simulink library "amg_high_precision_rtc"  (R2015b)
settings: Solver=ode45  StartTime=0.0  StopTime=10.0  RelTol=1e-3
libraries: simulink x207, waijung_soft_i2c_lib x11, amg_high_precision_rtc x10
(part 2 of 5)

== system amg_high_precision_rtc/STM32F4/DS3231 Get Date/Convert ==
  In1 : Inport
  In2 : Inport  Port=2
  In3 : Inport  Port=3
  In4 : Inport  Port=4
  Enable : EnablePort  PropagateVarSize=During execution
  Convert 1 : Subsystem
  Convert 2 : Subsystem
  Convert 3 : Subsystem
  Data Type Conversion{,1..3} (4 alike) : DataTypeConversion  OutDataTypeStr=uint8
  Extract Bits : simulink/Logic and Bit Operations/Extract Bits  SystemSampleTime=-1  bitsToExtract=Range of bits  numBits=8  bitIdxRange=[0 3]  outScalingMode=Treat bit field as an integer
  Day : Outport
  Date : Outport  Port=2
  Month : Outport  Port=3
  Year : Outport  Port=4
  wires:
  In1/1 -> Extract Bits/1
  Extract Bits/1 -> Data Type Conversion/1
  Convert 1/1(Out1) -> Data Type Conversion1/1
  In2/1 -> Convert 1/1(In1)
  In3/1 -> Convert 2/1(In1)
  Convert 2/1(Out1) -> Data Type Conversion2/1
  In4/1 -> Convert 3/1(In1)
  Convert 3/1(Out1) -> Data Type Conversion3/1
  Data Type Conversion/1 -> Day/1
  Data Type Conversion1/1 -> Date/1
  Data Type Conversion2/1 -> Month/1
  Data Type Conversion3/1 -> Year/1

== system amg_high_precision_rtc/STM32F4/DS3231 Get Time/Convert ==
  In1 : Inport
  In2 : Inport  Port=2
  In3 : Inport  Port=3
  Enable : EnablePort  PropagateVarSize=During execution
  Convert Hour : Subsystem
  Convert Second/ Minute : Subsystem
  Demux : Demux  Outputs=2
  Mux : Mux  Inputs=2
  Hour : Outport
  Minute : Outport  Port=2
  Second : Outport  Port=3
  AM/PM : Outport  Port=4
  wires:
  In2/1 -> Mux/2
  In1/1 -> Mux/1
  Mux/1 -> Convert Second/ Minute/1(In1)
  Convert Second/ Minute/1(Out1) -> Demux/1
  Demux/1 -> Second/1
  Demux/2 -> Minute/1
  In3/1 -> Convert Hour/1(In1)
  Convert Hour/1(Hour) -> Hour/1
  Convert Hour/2(AM/PM) -> AM/PM/1

== system amg_high_precision_rtc/STM32F4/DS3231 Set Date/ConvertToBCD1 ==
  In1 : Inport
  Bitwise Operator : simulink/Logic and Bit Operations/Bitwise Operator  logicop=OR  UseBitMask=off  NumInputPorts=2  BitMask=bin2dec('11011001')  BitMaskRealWorld=Stored Integer
  Constant : Constant  Value=10  OutDataTypeStr=single
  Constant1 : Constant  Value=10  OutDataTypeStr=single
  Data Type Conversion : DataTypeConversion  OutDataTypeStr=single
  Data Type Conversion1 : DataTypeConversion  OutDataTypeStr=uint8
  Data Type Conversion2 : DataTypeConversion  OutDataTypeStr=uint8
  Data Type Conversion3 : DataTypeConversion  OutDataTypeStr=uint8
  Divide : Product  Inputs=*/
  Product : Product  RndMeth=Zero
  Shift Arithmetic : simulink/Logic and Bit Operations/Shift Arithmetic  SystemSampleTime=-1  nBitShiftRight=-4  nBinPtShiftRight=0
  Subtract : Sum  Inputs=+-
  Out1 : Outport
  wires:
  Bitwise Operator/1 -> Out1/1
  Data Type Conversion3/1 -> Bitwise Operator/2
  Data Type Conversion2/1 -> Bitwise Operator/1
  Shift Arithmetic/1 -> Data Type Conversion3/1
  Subtract/1 -> Data Type Conversion2/1
  Constant1/1 -> Product/1
  Product/1 -> Subtract/2
  Data Type Conversion1/1 -> Shift Arithmetic/1, Product/2
  Divide/1 -> Data Type Conversion1/1
  Data Type Conversion/1 -> Divide/1
  In1/1 -> Subtract/1, Data Type Conversion/1
  Constant/1 -> Divide/2

== system amg_high_precision_rtc/STM32F4/DS3231 Set Date/ConvertToBCD2 ==
  In1 : Inport
  Bitwise Operator : simulink/Logic and Bit Operations/Bitwise Operator  logicop=OR  UseBitMask=off  NumInputPorts=2  BitMask=bin2dec('11011001')  BitMaskRealWorld=Stored Integer
  Constant : Constant  Value=10  OutDataTypeStr=single
  Constant1 : Constant  Value=10  OutDataTypeStr=single
  Data Type Conversion : DataTypeConversion  OutDataTypeStr=single
  Data Type Conversion1 : DataTypeConversion  OutDataTypeStr=uint8
  Data Type Conversion2 : DataTypeConversion  OutDataTypeStr=uint8
  Data Type Conversion3 : DataTypeConversion  OutDataTypeStr=uint8
  Divide : Product  Inputs=*/
  Product : Product  RndMeth=Zero
  Shift Arithmetic : simulink/Logic and Bit Operations/Shift Arithmetic  SystemSampleTime=-1  nBitShiftRight=-4  nBinPtShiftRight=0
  Subtract : Sum  Inputs=+-
  Out1 : Outport
  wires:
  Constant/1 -> Divide/2
  In1/1 -> Data Type Conversion/1, Subtract/1
  Data Type Conversion/1 -> Divide/1
  Divide/1 -> Data Type Conversion1/1
  Data Type Conversion1/1 -> Product/2, Shift Arithmetic/1
  Product/1 -> Subtract/2
  Constant1/1 -> Product/1
  Subtract/1 -> Data Type Conversion2/1
  Shift Arithmetic/1 -> Data Type Conversion3/1
  Data Type Conversion2/1 -> Bitwise Operator/1
  Data Type Conversion3/1 -> Bitwise Operator/2
  Bitwise Operator/1 -> Out1/1

== system amg_high_precision_rtc/STM32F4/DS3231 Set Date/ConvertToBCD3 ==
  In1 : Inport
  Bitwise Operator : simulink/Logic and Bit Operations/Bitwise Operator  logicop=OR  UseBitMask=off  NumInputPorts=2  BitMask=bin2dec('11011001')  BitMaskRealWorld=Stored Integer
  Constant : Constant  Value=10  OutDataTypeStr=single
  Constant1 : Constant  Value=10  OutDataTypeStr=single
  Data Type Conversion : DataTypeConversion  OutDataTypeStr=single
  Data Type Conversion1 : DataTypeConversion  OutDataTypeStr=uint8
  Data Type Conversion2 : DataTypeConversion  OutDataTypeStr=uint8
  Data Type Conversion3 : DataTypeConversion  OutDataTypeStr=uint8
  Divide : Product  Inputs=*/
  Product : Product  RndMeth=Zero
  Shift Arithmetic : simulink/Logic and Bit Operations/Shift Arithmetic  SystemSampleTime=-1  nBitShiftRight=-4  nBinPtShiftRight=0
  Subtract : Sum  Inputs=+-
  Out1 : Outport
  wires:
  Constant/1 -> Divide/2
  In1/1 -> Data Type Conversion/1, Subtract/1
  Data Type Conversion/1 -> Divide/1
  Divide/1 -> Data Type Conversion1/1
  Data Type Conversion1/1 -> Product/2, Shift Arithmetic/1
  Product/1 -> Subtract/2
  Constant1/1 -> Product/1
  Subtract/1 -> Data Type Conversion2/1
  Shift Arithmetic/1 -> Data Type Conversion3/1
  Data Type Conversion2/1 -> Bitwise Operator/1
  Data Type Conversion3/1 -> Bitwise Operator/2
  Bitwise Operator/1 -> Out1/1

== system amg_high_precision_rtc/STM32F4/DS3231 Set Time/ConvertToBCD1 ==
  In1 : Inport
  Bitwise Operator : simulink/Logic and Bit Operations/Bitwise Operator  logicop=OR  UseBitMask=off  NumInputPorts=2  BitMask=bin2dec('11011001')  BitMaskRealWorld=Stored Integer
  Constant : Constant  Value=10  OutDataTypeStr=single
  Constant1 : Constant  Value=10  OutDataTypeStr=single
  Data Type Conversion : DataTypeConversion  OutDataTypeStr=single
  Data Type Conversion1 : DataTypeConversion  OutDataTypeStr=uint8
  Data Type Conversion2 : DataTypeConversion  OutDataTypeStr=uint8
  Data Type Conversion3 : DataTypeConversion  OutDataTypeStr=uint8
  Divide : Product  Inputs=*/
  Product : Product  RndMeth=Zero
  Shift Arithmetic : simulink/Logic and Bit Operations/Shift Arithmetic  SystemSampleTime=-1  nBitShiftRight=-4  nBinPtShiftRight=0
  Subtract : Sum  Inputs=+-
  Out1 : Outport
  wires:
  Bitwise Operator/1 -> Out1/1
  Data Type Conversion3/1 -> Bitwise Operator/2
  Data Type Conversion2/1 -> Bitwise Operator/1
  Shift Arithmetic/1 -> Data Type Conversion3/1
  Subtract/1 -> Data Type Conversion2/1
  Constant1/1 -> Product/1
  Product/1 -> Subtract/2
  Data Type Conversion1/1 -> Shift Arithmetic/1, Product/2
  Divide/1 -> Data Type Conversion1/1
  Data Type Conversion/1 -> Divide/1
  In1/1 -> Subtract/1, Data Type Conversion/1
  Constant/1 -> Divide/2

== system amg_high_precision_rtc/STM32F4/DS3231 Set Time/ConvertToBCD2 ==
  In1 : Inport
  Bitwise Operator : simulink/Logic and Bit Operations/Bitwise Operator  logicop=OR  UseBitMask=off  NumInputPorts=2  BitMask=bin2dec('11011001')  BitMaskRealWorld=Stored Integer
  Constant : Constant  Value=10  OutDataTypeStr=single
  Constant1 : Constant  Value=10  OutDataTypeStr=single
  Data Type Conversion : DataTypeConversion  OutDataTypeStr=single
  Data Type Conversion1 : DataTypeConversion  OutDataTypeStr=uint8
  Data Type Conversion2 : DataTypeConversion  OutDataTypeStr=uint8
  Data Type Conversion3 : DataTypeConversion  OutDataTypeStr=uint8
  Divide : Product  Inputs=*/
  Product : Product  RndMeth=Zero
  Shift Arithmetic : simulink/Logic and Bit Operations/Shift Arithmetic  SystemSampleTime=-1  nBitShiftRight=-4  nBinPtShiftRight=0
  Subtract : Sum  Inputs=+-
  Out1 : Outport
  wires:
  Constant/1 -> Divide/2
  In1/1 -> Data Type Conversion/1, Subtract/1
  Data Type Conversion/1 -> Divide/1
  Divide/1 -> Data Type Conversion1/1
  Data Type Conversion1/1 -> Product/2, Shift Arithmetic/1
  Product/1 -> Subtract/2
  Constant1/1 -> Product/1
  Subtract/1 -> Data Type Conversion2/1
  Shift Arithmetic/1 -> Data Type Conversion3/1
  Data Type Conversion2/1 -> Bitwise Operator/1
  Data Type Conversion3/1 -> Bitwise Operator/2
  Bitwise Operator/1 -> Out1/1

== system amg_high_precision_rtc/STM32F4/DS3231 Set Time/ConvertToBCD3 ==
  In1 : Inport
  Bitwise Operator : simulink/Logic and Bit Operations/Bitwise Operator  logicop=OR  UseBitMask=off  NumInputPorts=2  BitMask=bin2dec('11011001')  BitMaskRealWorld=Stored Integer
  Constant : Constant  Value=10  OutDataTypeStr=single
  Constant1 : Constant  Value=10  OutDataTypeStr=single
  Data Type Conversion : DataTypeConversion  OutDataTypeStr=single
  Data Type Conversion1 : DataTypeConversion  OutDataTypeStr=uint8
  Data Type Conversion2 : DataTypeConversion  OutDataTypeStr=uint8
  Data Type Conversion3 : DataTypeConversion  OutDataTypeStr=uint8
  Divide : Product  Inputs=*/
  Product : Product  RndMeth=Zero
  Shift Arithmetic : simulink/Logic and Bit Operations/Shift Arithmetic  SystemSampleTime=-1  nBitShiftRight=-4  nBinPtShiftRight=0
  Subtract : Sum  Inputs=+-
  Out1 : Outport
  wires:
  Constant/1 -> Divide/2
  In1/1 -> Data Type Conversion/1, Subtract/1
  Data Type Conversion/1 -> Divide/1
  Divide/1 -> Data Type Conversion1/1
  Data Type Conversion1/1 -> Product/2, Shift Arithmetic/1
  Product/1 -> Subtract/2
  Constant1/1 -> Product/1
  Subtract/1 -> Data Type Conversion2/1
  Shift Arithmetic/1 -> Data Type Conversion3/1
  Data Type Conversion2/1 -> Bitwise Operator/1
  Data Type Conversion3/1 -> Bitwise Operator/2
  Bitwise Operator/1 -> Out1/1

== system amg_high_precision_rtc/STM32F4/DS3231Temperture/Check Busy// Write Conv ==
  In1 : Inport
  Enable : EnablePort  PropagateVarSize=During execution
  Bitwise Operator : simulink/Logic and Bit Operations/Bitwise Operator  logicop=AND  UseBitMask=on  BitMask=hex2dec('04')  BitMaskRealWorld=Stored Integer
  I2C Master Read/Write1 : S-Function  FunctionName=stm32f4_i2c  Parameters=configuration,module,transfer,clkspeed,timeout,sdapin,sclpin,writecount,readcount,inputtypearray,outputtypearray,confstr,sampletime,sampletimestr,blockid  SFunctionDeploymentMode=off  EnableBusSupport=off  mask(stm32f4_i2c){configuration=Transaction, module=1, lastmodule=3, transfer=Blocking, dutycycle=TLow/THigh = 2, clkspeed=400, timeout=25, writecount=1, readcount=1, sdapin=C9, sclpin=A8, waitwritetime=0, inputtypearray=[2 3 3], outputtypearray=[2 3 3], confstr=["C","9","A","8","1","1","6","0","I2C_DutyCycle_2","0"], sampletime=-1, sampletimestr=0, blockid=amg_high_precision_rtcTempertureReadI2CMasterReadWrite1}
      mask prompts: module "I2C Module"; lastmodule "Last module"; transfer "Transfer mode"; dutycycle "Duty cycle in fast mode"; clkspeed "Clock speed (kHz)"; timeout "Timeout (ms)"; writecount "Bytes write count"; readcount "Bytes read count"; sdapin "SDA pin"; sclpin "SCL pin"; waitwritetime "Wait write time (ms), default is 0"; inputtypearray "Input type array"; outputtypearray "Output type array"; confstr "Configuration string"; sampletime "Sample time (sec)"; sampletimestr "Compiled sample time (sec) in string"
      mask init:
      | stm32f4_i2c_callback('init');
      mask Help: web(fullfile(waijungdocroot,'stm32f4_i2c_readwrite.htm'), '-browser')
      mask TypeOptions configuration: Setup | Transaction
      mask Callback configuration: stm32f4_i2c_callback('configuration');
      mask TypeOptions module: 1 | 2 | 3
      mask Callback module: stm32f4_i2c_callback('module');
      mask TypeOptions transfer: Blocking | Non-blocking
      mask TypeOptions dutycycle: TLow/THigh = 16/9 | TLow/THigh = 2
      mask Callback dutycycle: stm32f4_i2c_callback('dutycycle');
      mask Callback writecount: stm32f4_i2c_callback('writecount');
      mask Callback readcount: stm32f4_i2c_callback('readcount');
      mask TypeOptions sdapin: - | C9
      mask Callback sdapin: stm32f4_i2c_callback('sdapin');
      mask TypeOptions sclpin: - | A8
      mask Callback sclpin: stm32f4_i2c_callback('sclpin');
      mask Callback confstr: stm32f4_i2c_callback('confstr');
      mask Callback sampletime: stm32f4_i2c_callback('sampletime');
      mask Callback sampletimestr: stm32f4_i2c_callback('sampletimestr');
      mask Callback blockid: stm32f4_i2c_callback('blockid');
      mask Display: text(0.5, 0.5, 'Module: I2C1\nTransfer: Blocking\nWrite: 1 bytes\nRead: 1 bytes\nTs (sec): 0','ver','middle','hor','center');port_label('input', 1,'SlvAddr');port_label('input', 2,'Wr0 (uint8)');port_label('output', 1,'Status');port_label('output', 2,'Rd0 (uint8)');
  If : If  NumInputs=2  IfExpression=(u1 == 0) & (u2 == 0)  ShowElse=off
  If Action Active CONV : Subsystem  TreatAsAtomicUnit=on
  REG_STA : Constant  Value=hex2dec('0F')  OutDataTypeStr=uint8
  wires:
  REG_STA/1 -> I2C Master Read/Write1/2
  I2C Master Read/Write1/1 -> If/1
  In1/1 -> I2C Master Read/Write1/1, If Action Active CONV/1(In1)
  I2C Master Read/Write1/2 -> Bitwise Operator/1
  Bitwise Operator/1 -> If/2
  If/1 -> If Action Active CONV/Action

== system amg_high_precision_rtc/STM32F4/DS3231Temperture/Convert ==
  In1 : Inport
  In2 : Inport  Port=2
  Enable : EnablePort  PropagateVarSize=During execution
  Bitwise Operator : simulink/Logic and Bit Operations/Bitwise Operator  logicop=OR  UseBitMask=off  NumInputPorts=2  BitMask=bin2dec('11011001')  BitMaskRealWorld=Stored Integer
  Constant : Constant  Value=single(0.25)
  Data Type Conversion : DataTypeConversion  OutDataTypeStr=uint16
  Data Type Conversion1 : DataTypeConversion  OutDataTypeStr=uint16
  Data Type Conversion2 : DataTypeConversion  OutDataTypeStr=int16
  Product : Product  OutDataTypeStr=single  RndMeth=Zero
  Shift Arithmetic1 : simulink/Logic and Bit Operations/Shift Arithmetic  SystemSampleTime=-1  nBitShiftRight=-8  nBinPtShiftRight=0
  Shift Arithmetic2 : simulink/Logic and Bit Operations/Shift Arithmetic  SystemSampleTime=-1  nBitShiftRight=6  nBinPtShiftRight=0
  Reading : Outport
  wires:
  In1/1 -> Data Type Conversion/1
  In2/1 -> Data Type Conversion1/1
  Data Type Conversion/1 -> Shift Arithmetic1/1
  Shift Arithmetic1/1 -> Bitwise Operator/1
  Data Type Conversion1/1 -> Bitwise Operator/2
  Bitwise Operator/1 -> Shift Arithmetic2/1
  Data Type Conversion2/1 -> Product/1
  Constant/1 -> Product/2
  Product/1 -> Reading/1
  Shift Arithmetic2/1 -> Data Type Conversion2/1

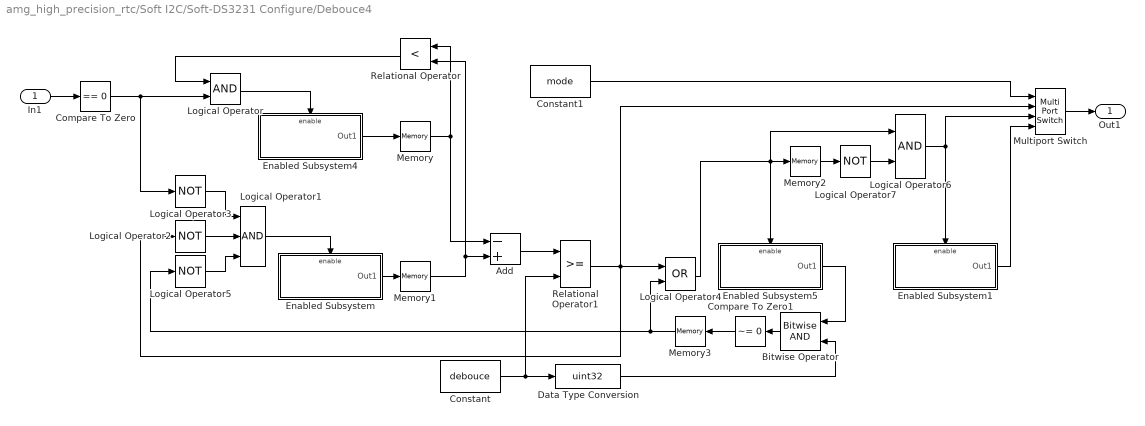
== system amg_high_precision_rtc/Soft I2C/Soft-DS3231 Configure/Debouce4 ==
  In1 : Inport
  Add : Sum  Inputs=-+  OutDataTypeStr=int32
  Bitwise Operator : simulink/Logic and Bit Operations/Bitwise Operator  logicop=AND  UseBitMask=off  NumInputPorts=2  BitMask=debouce  BitMaskRealWorld=Stored Integer
  Compare To Zero : simulink/Logic and Bit Operations/Compare To Zero  SystemSampleTime=-1  relop===  LogicOutDataTypeMode=uint8  ZeroCross=off
  Compare To Zero1 : simulink/Logic and Bit Operations/Compare To Zero  SystemSampleTime=-1  relop=~=  LogicOutDataTypeMode=boolean  ZeroCross=off
  Constant : Constant  Value=debouce  OutDataTypeStr=int32
  Constant1 : Constant  Value=mode  OutDataTypeStr=int32
  Data Type Conversion : DataTypeConversion  OutDataTypeStr=uint32
  Enabled Subsystem : Subsystem  TreatAsAtomicUnit=on
  Enabled Subsystem1 : Subsystem  TreatAsAtomicUnit=on
  Enabled Subsystem4 : Subsystem  TreatAsAtomicUnit=on
  Enabled Subsystem5 : Subsystem  TreatAsAtomicUnit=on
  Logical Operator : Logic  AllPortsSameDT=off  OutDataTypeStr=boolean
  Logical Operator1 : Logic  Inputs=3  AllPortsSameDT=off  OutDataTypeStr=boolean
  Logical Operator{2..3,5,7} (4 alike) : Logic  Operator=NOT  AllPortsSameDT=off  OutDataTypeStr=boolean
  Logical Operator4 : Logic  Operator=OR  AllPortsSameDT=off  OutDataTypeStr=boolean
  Logical Operator6 : Logic  AllPortsSameDT=off  OutDataTypeStr=boolean
  Memory{,1..3} (4 alike) : Memory  LinearizeMemory=on
  Multiport Switch : MultiPortSwitch
  Relational Operator : RelationalOperator  Operator=<  OutDataTypeStr=boolean
  Relational Operator1 : RelationalOperator  OutDataTypeStr=boolean  InputSameDT=on
  Out1 : Outport
  wires:
  Logical Operator1/1 -> Enabled Subsystem/Enable
  Relational Operator1/1 -> Logical Operator2/1, Logical Operator4/1, Multiport Switch/2
  Logical Operator7/1 -> Logical Operator6/2
  Memory2/1 -> Logical Operator7/1
  Logical Operator4/1 -> Logical Operator6/1, Memory2/1, Enabled Subsystem5/Enable
  Enabled Subsystem5/1(Out1) -> Bitwise Operator/1
  Bitwise Operator/1 -> Compare To Zero1/1
  Compare To Zero1/1 -> Memory3/1
  Logical Operator3/1 -> Logical Operator1/1
  Logical Operator5/1 -> Logical Operator1/3
  Memory3/1 -> Logical Operator5/1, Logical Operator4/2
  Logical Operator2/1 -> Logical Operator1/2
  Constant/1 -> Relational Operator1/2, Data Type Conversion/1
  Add/1 -> Relational Operator1/1
  Relational Operator/1 -> Logical Operator/1
  Logical Operator/1 -> Enabled Subsystem4/Enable
  Compare To Zero/1 -> Logical Operator3/1, Logical Operator/2
  Memory1/1 -> Relational Operator/2, Add/2
  Memory/1 -> Add/1, Relational Operator/1
  Enabled Subsystem4/1(Out1) -> Memory/1
  Enabled Subsystem/1(Out1) -> Memory1/1
  In1/1 -> Compare To Zero/1
  Logical Operator6/1 -> Multiport Switch/3, Enabled Subsystem1/Enable
  Enabled Subsystem1/1(Out1) -> Multiport Switch/4
  Data Type Conversion/1 -> Bitwise Operator/2
  Multiport Switch/1 -> Out1/1
  Constant1/1 -> Multiport Switch/1

== system amg_high_precision_rtc/Soft I2C/Soft-DS3231 Configure/Enabled Subsystem ==
  note: # Mode ID
      | 0 - DD
      | 1 - MM
      | 2 - YY
      | 3 - HH
      | 4 - MM
      | 5 - SS
  SlvAddr : Inport
  UP : Inport  Port=2
  DOWN : Inport  Port=3
  MODE : Inport  Port=4
  Enable : EnablePort  PropagateVarSize=During execution
  Debouce1 : Subsystem  TreatAsAtomicUnit=on  mask{mode=Single Pulse, prescale=4, debouce=7}
      mask prompts: prescale "Prescale (Debouce count)"; debouce "Debouce value"
      settings: RTWFcnNameOpts=Use subsystem name  RTWFileNameOpts=Use function name
      mask TypeOptions mode: Normal | Single Pulse | Toggle Latch
      mask Callback mode: waijung_intput_validation_callback('mode');
      mask TypeOptions prescale: 4 | 8 | 16 | 32 | 64 | 128 | 256 | 512 | 1024 | 2048 | 4096 | 8192
      mask Callback debouce: waijung_intput_validation_callback('prescale');
      mask Display: disp('Button Pressed\n(Single Pulse)\nDebounce count: 4');
  Debouce2 : Subsystem  TreatAsAtomicUnit=on  mask{mode=Single Pulse, prescale=4, debouce=3}
      mask prompts: prescale "Prescale (Debouce count)"; debouce "Debouce value"
      settings: RTWFcnNameOpts=Use subsystem name  RTWFileNameOpts=Use function name
      mask TypeOptions mode: Normal | Single Pulse | Toggle Latch
      mask Callback mode: waijung_intput_validation_callback('mode');
      mask TypeOptions prescale: 4 | 8 | 16 | 32 | 64 | 128 | 256 | 512 | 1024 | 2048 | 4096 | 8192
      mask Callback debouce: waijung_intput_validation_callback('prescale');
      mask Display: disp('Button Pressed\n(Single Pulse)\nDebounce count: 4');
  Debouce3 : Subsystem  TreatAsAtomicUnit=on  mask{mode=Single Pulse, prescale=4, debouce=3}
      mask prompts: prescale "Prescale (Debouce count)"; debouce "Debouce value"
      settings: RTWFcnNameOpts=Use subsystem name  RTWFileNameOpts=Use function name
      mask TypeOptions mode: Normal | Single Pulse | Toggle Latch
      mask Callback mode: waijung_intput_validation_callback('mode');
      mask TypeOptions prescale: 4 | 8 | 16 | 32 | 64 | 128 | 256 | 512 | 1024 | 2048 | 4096 | 8192
      mask Callback debouce: waijung_intput_validation_callback('prescale');
      mask Display: disp('Button Pressed\n(Single Pulse)\nDebounce count: 4');
  Generate Mode ID : Subsystem
  Logical Operator : Logic  Operator=OR  AllPortsSameDT=off  OutDataTypeStr=boolean
  Subsystem : Subsystem
  Adjust state : Outport
  wires:
  SlvAddr/1 -> Subsystem/3(SlvAddr)
  Logical Operator/1 -> Subsystem/Enable
  Debouce2/1(Out1) -> Subsystem/1(Up), Logical Operator/1
  Debouce3/1(Out1) -> Subsystem/2(Down), Logical Operator/2
  Generate Mode ID/1(Out1) -> Subsystem/4(Adjust State), Adjust state/1
  Debouce1/1(Out1) -> Generate Mode ID/1(In1)
  MODE/1 -> Debouce1/1(In1)
  DOWN/1 -> Debouce3/1(In1)
  UP/1 -> Debouce2/1(In1)

== system amg_high_precision_rtc/Soft I2C/Soft-DS3231 Get Date/Convert ==
  In1 : Inport
  In2 : Inport  Port=2
  In3 : Inport  Port=3
  In4 : Inport  Port=4
  Enable : EnablePort  PropagateVarSize=During execution
  Convert 1 : Subsystem
  Convert 2 : Subsystem
  Convert 3 : Subsystem
  Data Type Conversion{,1..3} (4 alike) : DataTypeConversion  OutDataTypeStr=uint8
  Extract Bits : simulink/Logic and Bit Operations/Extract Bits  SystemSampleTime=-1  bitsToExtract=Range of bits  numBits=8  bitIdxRange=[0 3]  outScalingMode=Treat bit field as an integer
  Day : Outport
  Date : Outport  Port=2
  Month : Outport  Port=3
  Year : Outport  Port=4
  wires:
  Data Type Conversion3/1 -> Year/1
  Data Type Conversion2/1 -> Month/1
  Data Type Conversion1/1 -> Date/1
  Data Type Conversion/1 -> Day/1
  Convert 3/1(Out1) -> Data Type Conversion3/1
  In4/1 -> Convert 3/1(In1)
  Convert 2/1(Out1) -> Data Type Conversion2/1
  In3/1 -> Convert 2/1(In1)
  In2/1 -> Convert 1/1(In1)
  Convert 1/1(Out1) -> Data Type Conversion1/1
  Extract Bits/1 -> Data Type Conversion/1
  In1/1 -> Extract Bits/1

== system amg_high_precision_rtc/Soft I2C/Soft-DS3231 Get Time/Convert ==
  In1 : Inport
  In2 : Inport  Port=2
  In3 : Inport  Port=3
  Enable : EnablePort  PropagateVarSize=During execution
  Convert Hour : Subsystem
  Convert Second/ Minute : Subsystem
  Demux : Demux  Outputs=2
  Mux : Mux  Inputs=2
  Hour : Outport
  Minute : Outport  Port=2
  Second : Outport  Port=3
  AM/PM : Outport  Port=4
  wires:
  Convert Hour/2(AM/PM) -> AM/PM/1
  Convert Hour/1(Hour) -> Hour/1
  In3/1 -> Convert Hour/1(In1)
  Demux/2 -> Minute/1
  Demux/1 -> Second/1
  Convert Second/ Minute/1(Out1) -> Demux/1
  Mux/1 -> Convert Second/ Minute/1(In1)
  In1/1 -> Mux/1
  In2/1 -> Mux/2

== system amg_high_precision_rtc/Soft I2C/Soft-DS3231 Set Date/ConvertToBCD1 ==
  In1 : Inport
  Bitwise Operator : simulink/Logic and Bit Operations/Bitwise Operator  logicop=OR  UseBitMask=off  NumInputPorts=2  BitMask=bin2dec('11011001')  BitMaskRealWorld=Stored Integer
  Constant : Constant  Value=10  OutDataTypeStr=single
  Constant1 : Constant  Value=10  OutDataTypeStr=single
  Data Type Conversion : DataTypeConversion  OutDataTypeStr=single
  Data Type Conversion1 : DataTypeConversion  OutDataTypeStr=uint8
  Data Type Conversion2 : DataTypeConversion  OutDataTypeStr=uint8
  Data Type Conversion3 : DataTypeConversion  OutDataTypeStr=uint8
  Divide : Product  Inputs=*/
  Product : Product  RndMeth=Zero
  Shift Arithmetic : simulink/Logic and Bit Operations/Shift Arithmetic  SystemSampleTime=-1  nBitShiftRight=-4  nBinPtShiftRight=0
  Subtract : Sum  Inputs=+-
  Out1 : Outport
  wires:
  Constant/1 -> Divide/2
  In1/1 -> Data Type Conversion/1, Subtract/1
  Data Type Conversion/1 -> Divide/1
  Divide/1 -> Data Type Conversion1/1
  Data Type Conversion1/1 -> Product/2, Shift Arithmetic/1
  Product/1 -> Subtract/2
  Constant1/1 -> Product/1
  Subtract/1 -> Data Type Conversion2/1
  Shift Arithmetic/1 -> Data Type Conversion3/1
  Data Type Conversion2/1 -> Bitwise Operator/1
  Data Type Conversion3/1 -> Bitwise Operator/2
  Bitwise Operator/1 -> Out1/1

== system amg_high_precision_rtc/Soft I2C/Soft-DS3231 Set Date/ConvertToBCD2 ==
  In1 : Inport
  Bitwise Operator : simulink/Logic and Bit Operations/Bitwise Operator  logicop=OR  UseBitMask=off  NumInputPorts=2  BitMask=bin2dec('11011001')  BitMaskRealWorld=Stored Integer
  Constant : Constant  Value=10  OutDataTypeStr=single
  Constant1 : Constant  Value=10  OutDataTypeStr=single
  Data Type Conversion : DataTypeConversion  OutDataTypeStr=single
  Data Type Conversion1 : DataTypeConversion  OutDataTypeStr=uint8
  Data Type Conversion2 : DataTypeConversion  OutDataTypeStr=uint8
  Data Type Conversion3 : DataTypeConversion  OutDataTypeStr=uint8
  Divide : Product  Inputs=*/
  Product : Product  RndMeth=Zero
  Shift Arithmetic : simulink/Logic and Bit Operations/Shift Arithmetic  SystemSampleTime=-1  nBitShiftRight=-4  nBinPtShiftRight=0
  Subtract : Sum  Inputs=+-
  Out1 : Outport
  wires:
  Bitwise Operator/1 -> Out1/1
  Data Type Conversion3/1 -> Bitwise Operator/2
  Data Type Conversion2/1 -> Bitwise Operator/1
  Shift Arithmetic/1 -> Data Type Conversion3/1
  Subtract/1 -> Data Type Conversion2/1
  Constant1/1 -> Product/1
  Product/1 -> Subtract/2
  Data Type Conversion1/1 -> Shift Arithmetic/1, Product/2
  Divide/1 -> Data Type Conversion1/1
  Data Type Conversion/1 -> Divide/1
  In1/1 -> Subtract/1, Data Type Conversion/1
  Constant/1 -> Divide/2

== system amg_high_precision_rtc/Soft I2C/Soft-DS3231 Set Date/ConvertToBCD3 ==
  In1 : Inport
  Bitwise Operator : simulink/Logic and Bit Operations/Bitwise Operator  logicop=OR  UseBitMask=off  NumInputPorts=2  BitMask=bin2dec('11011001')  BitMaskRealWorld=Stored Integer
  Constant : Constant  Value=10  OutDataTypeStr=single
  Constant1 : Constant  Value=10  OutDataTypeStr=single
  Data Type Conversion : DataTypeConversion  OutDataTypeStr=single
  Data Type Conversion1 : DataTypeConversion  OutDataTypeStr=uint8
  Data Type Conversion2 : DataTypeConversion  OutDataTypeStr=uint8
  Data Type Conversion3 : DataTypeConversion  OutDataTypeStr=uint8
  Divide : Product  Inputs=*/
  Product : Product  RndMeth=Zero
  Shift Arithmetic : simulink/Logic and Bit Operations/Shift Arithmetic  SystemSampleTime=-1  nBitShiftRight=-4  nBinPtShiftRight=0
  Subtract : Sum  Inputs=+-
  Out1 : Outport
  wires:
  Bitwise Operator/1 -> Out1/1
  Data Type Conversion3/1 -> Bitwise Operator/2
  Data Type Conversion2/1 -> Bitwise Operator/1
  Shift Arithmetic/1 -> Data Type Conversion3/1
  Subtract/1 -> Data Type Conversion2/1
  Constant1/1 -> Product/1
  Product/1 -> Subtract/2
  Data Type Conversion1/1 -> Shift Arithmetic/1, Product/2
  Divide/1 -> Data Type Conversion1/1
  Data Type Conversion/1 -> Divide/1
  In1/1 -> Subtract/1, Data Type Conversion/1
  Constant/1 -> Divide/2

== system amg_high_precision_rtc/Soft I2C/Soft-DS3231 Set Time/ConvertToBCD1 ==
  In1 : Inport
  Bitwise Operator : simulink/Logic and Bit Operations/Bitwise Operator  logicop=OR  UseBitMask=off  NumInputPorts=2  BitMask=bin2dec('11011001')  BitMaskRealWorld=Stored Integer
  Constant : Constant  Value=10  OutDataTypeStr=single
  Constant1 : Constant  Value=10  OutDataTypeStr=single
  Data Type Conversion : DataTypeConversion  OutDataTypeStr=single
  Data Type Conversion1 : DataTypeConversion  OutDataTypeStr=uint8
  Data Type Conversion2 : DataTypeConversion  OutDataTypeStr=uint8
  Data Type Conversion3 : DataTypeConversion  OutDataTypeStr=uint8
  Divide : Product  Inputs=*/
  Product : Product  RndMeth=Zero
  Shift Arithmetic : simulink/Logic and Bit Operations/Shift Arithmetic  SystemSampleTime=-1  nBitShiftRight=-4  nBinPtShiftRight=0
  Subtract : Sum  Inputs=+-
  Out1 : Outport
  wires:
  Constant/1 -> Divide/2
  In1/1 -> Data Type Conversion/1, Subtract/1
  Data Type Conversion/1 -> Divide/1
  Divide/1 -> Data Type Conversion1/1
  Data Type Conversion1/1 -> Product/2, Shift Arithmetic/1
  Product/1 -> Subtract/2
  Constant1/1 -> Product/1
  Subtract/1 -> Data Type Conversion2/1
  Shift Arithmetic/1 -> Data Type Conversion3/1
  Data Type Conversion2/1 -> Bitwise Operator/1
  Data Type Conversion3/1 -> Bitwise Operator/2
  Bitwise Operator/1 -> Out1/1

== system amg_high_precision_rtc/Soft I2C/Soft-DS3231 Set Time/ConvertToBCD2 ==
  In1 : Inport
  Bitwise Operator : simulink/Logic and Bit Operations/Bitwise Operator  logicop=OR  UseBitMask=off  NumInputPorts=2  BitMask=bin2dec('11011001')  BitMaskRealWorld=Stored Integer
  Constant : Constant  Value=10  OutDataTypeStr=single
  Constant1 : Constant  Value=10  OutDataTypeStr=single
  Data Type Conversion : DataTypeConversion  OutDataTypeStr=single
  Data Type Conversion1 : DataTypeConversion  OutDataTypeStr=uint8
  Data Type Conversion2 : DataTypeConversion  OutDataTypeStr=uint8
  Data Type Conversion3 : DataTypeConversion  OutDataTypeStr=uint8
  Divide : Product  Inputs=*/
  Product : Product  RndMeth=Zero
  Shift Arithmetic : simulink/Logic and Bit Operations/Shift Arithmetic  SystemSampleTime=-1  nBitShiftRight=-4  nBinPtShiftRight=0
  Subtract : Sum  Inputs=+-
  Out1 : Outport
  wires:
  Bitwise Operator/1 -> Out1/1
  Data Type Conversion3/1 -> Bitwise Operator/2
  Data Type Conversion2/1 -> Bitwise Operator/1
  Shift Arithmetic/1 -> Data Type Conversion3/1
  Subtract/1 -> Data Type Conversion2/1
  Constant1/1 -> Product/1
  Product/1 -> Subtract/2
  Data Type Conversion1/1 -> Shift Arithmetic/1, Product/2
  Divide/1 -> Data Type Conversion1/1
  Data Type Conversion/1 -> Divide/1
  In1/1 -> Subtract/1, Data Type Conversion/1
  Constant/1 -> Divide/2

== system amg_high_precision_rtc/Soft I2C/Soft-DS3231 Set Time/ConvertToBCD3 ==
  In1 : Inport
  Bitwise Operator : simulink/Logic and Bit Operations/Bitwise Operator  logicop=OR  UseBitMask=off  NumInputPorts=2  BitMask=bin2dec('11011001')  BitMaskRealWorld=Stored Integer
  Constant : Constant  Value=10  OutDataTypeStr=single
  Constant1 : Constant  Value=10  OutDataTypeStr=single
  Data Type Conversion : DataTypeConversion  OutDataTypeStr=single
  Data Type Conversion1 : DataTypeConversion  OutDataTypeStr=uint8
  Data Type Conversion2 : DataTypeConversion  OutDataTypeStr=uint8
  Data Type Conversion3 : DataTypeConversion  OutDataTypeStr=uint8
  Divide : Product  Inputs=*/
  Product : Product  RndMeth=Zero
  Shift Arithmetic : simulink/Logic and Bit Operations/Shift Arithmetic  SystemSampleTime=-1  nBitShiftRight=-4  nBinPtShiftRight=0
  Subtract : Sum  Inputs=+-
  Out1 : Outport
  wires:
  Bitwise Operator/1 -> Out1/1
  Data Type Conversion3/1 -> Bitwise Operator/2
  Data Type Conversion2/1 -> Bitwise Operator/1
  Shift Arithmetic/1 -> Data Type Conversion3/1
  Subtract/1 -> Data Type Conversion2/1
  Constant1/1 -> Product/1
  Product/1 -> Subtract/2
  Data Type Conversion1/1 -> Shift Arithmetic/1, Product/2
  Divide/1 -> Data Type Conversion1/1
  Data Type Conversion/1 -> Divide/1
  In1/1 -> Subtract/1, Data Type Conversion/1
  Constant/1 -> Divide/2

== system amg_high_precision_rtc/Soft I2C/Soft-DS3231Temperture/Check Busy// Write Conv ==
  In1 : Inport
  Enable : EnablePort  PropagateVarSize=During execution
  Bitwise Operator : simulink/Logic and Bit Operations/Bitwise Operator  logicop=AND  UseBitMask=on  BitMask=hex2dec('04')  BitMaskRealWorld=Stored Integer
  If : If  NumInputs=2  IfExpression=(u1 == 0) & (u2 == 0)  ShowElse=off
  If Action Active CONV : Subsystem  TreatAsAtomicUnit=on
  REG_STA : Constant  Value=hex2dec('0F')  OutDataTypeStr=uint8
  Soft I2C Master Read/Write : waijung_soft_i2c_lib/Soft I2C Master Read//Write  conf=ReadWrite  targetname=0  module=1  transfer=Blocking  clk=100  timeout=25  sdapins={'A4','A6'}  sclpins='A5'  writecount=1  readcount=1  waittime=0  forcestop=off  portpinstr=0  sampletime=-1  blockid=SoftI2CSoftDS3231TempertureCheckBusyWriteConvSoftI2CMasterReadWrite  inputporttype=[3 3]  inputportwidth=[]  inputportlabel={'SlvAddr' 'Wr0 (uint8)'}  outputporttype=[3 3 ]  outputportwidth=[1 1]  outputportlabel={'Status' 'Rd0 (uint8)'}  compat=0  optionstring=[]
  wires:
  Bitwise Operator/1 -> If/2
  Soft I2C Master Read/Write/2 -> Bitwise Operator/1
  In1/1 -> If Action Active CONV/1(In1), Soft I2C Master Read/Write/1
  Soft I2C Master Read/Write/1 -> If/1
  REG_STA/1 -> Soft I2C Master Read/Write/2
  If/1 -> If Action Active CONV/Action

== system amg_high_precision_rtc/Soft I2C/Soft-DS3231Temperture/Convert ==
  In1 : Inport
  In2 : Inport  Port=2
  Enable : EnablePort  PropagateVarSize=During execution
  Bitwise Operator : simulink/Logic and Bit Operations/Bitwise Operator  logicop=OR  UseBitMask=off  NumInputPorts=2  BitMask=bin2dec('11011001')  BitMaskRealWorld=Stored Integer
  Constant : Constant  Value=single(0.25)
  Data Type Conversion : DataTypeConversion  OutDataTypeStr=uint16
  Data Type Conversion1 : DataTypeConversion  OutDataTypeStr=uint16
  Data Type Conversion2 : DataTypeConversion  OutDataTypeStr=int16
  Product : Product  OutDataTypeStr=single  RndMeth=Zero
  Shift Arithmetic1 : simulink/Logic and Bit Operations/Shift Arithmetic  SystemSampleTime=-1  nBitShiftRight=-8  nBinPtShiftRight=0
  Shift Arithmetic2 : simulink/Logic and Bit Operations/Shift Arithmetic  SystemSampleTime=-1  nBitShiftRight=6  nBinPtShiftRight=0
  Reading : Outport
  wires:
  Shift Arithmetic2/1 -> Data Type Conversion2/1
  Product/1 -> Reading/1
  Constant/1 -> Product/2
  Data Type Conversion2/1 -> Product/1
  Bitwise Operator/1 -> Shift Arithmetic2/1
  Data Type Conversion1/1 -> Bitwise Operator/2
  Shift Arithmetic1/1 -> Bitwise Operator/1
  Data Type Conversion/1 -> Shift Arithmetic1/1
  In2/1 -> Data Type Conversion1/1
  In1/1 -> Data Type Conversion/1

== system amg_high_precision_rtc/STM32F4/DS3231 Configure/Debouce4/Enabled Subsystem ==
  Enable : EnablePort  PropagateVarSize=During execution
  Counter Free-Running : simulink/Sources/Counter Free-Running  SystemSampleTime=-1  NumBits=32  tsamp=-1
  Out1 : Outport  InitialOutput=0
  wires:
  Counter Free-Running/1 -> Out1/1

== system amg_high_precision_rtc/STM32F4/DS3231 Configure/Debouce4/Enabled Subsystem1 ==
  Enable : EnablePort  PropagateVarSize=During execution
  Bitwise Operator : simulink/Logic and Bit Operations/Bitwise Operator  logicop=AND  UseBitMask=on  BitMask=1  BitMaskRealWorld=Stored Integer
  Compare To Zero : simulink/Logic and Bit Operations/Compare To Zero  SystemSampleTime=-1  relop===  LogicOutDataTypeMode=uint8  ZeroCross=off
  Counter Free-Running : simulink/Sources/Counter Free-Running  SystemSampleTime=-1  NumBits=32  tsamp=-1
  Out1 : Outport  InitialOutput=0
  wires:
  Counter Free-Running/1 -> Bitwise Operator/1
  Bitwise Operator/1 -> Compare To Zero/1
  Compare To Zero/1 -> Out1/1

== system amg_high_precision_rtc/STM32F4/DS3231 Configure/Debouce4/Enabled Subsystem4 ==
  Enable : EnablePort  PropagateVarSize=During execution
  Counter Free-Running : simulink/Sources/Counter Free-Running  SystemSampleTime=-1  NumBits=32  tsamp=-1
  Out1 : Outport  InitialOutput=0
  wires:
  Counter Free-Running/1 -> Out1/1

== system amg_high_precision_rtc/STM32F4/DS3231 Configure/Debouce4/Enabled Subsystem5 ==
  Enable : EnablePort  PropagateVarSize=During execution
  Counter Free-Running : simulink/Sources/Counter Free-Running  SystemSampleTime=-1  NumBits=32  tsamp=-1
  Out1 : Outport  InitialOutput=0
  wires:
  Counter Free-Running/1 -> Out1/1

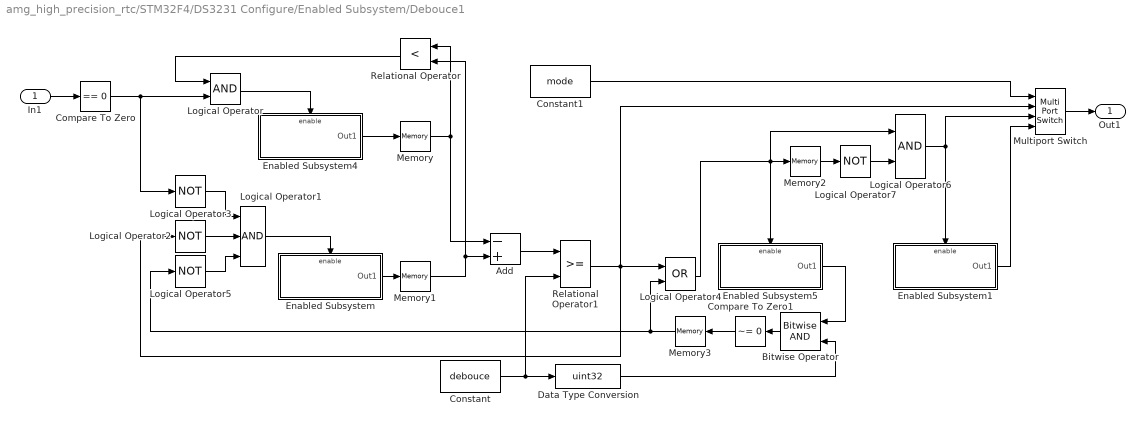
== system amg_high_precision_rtc/STM32F4/DS3231 Configure/Enabled Subsystem/Debouce1 ==
  In1 : Inport
  Add : Sum  Inputs=-+  OutDataTypeStr=int32
  Bitwise Operator : simulink/Logic and Bit Operations/Bitwise Operator  logicop=AND  UseBitMask=off  NumInputPorts=2  BitMask=debouce  BitMaskRealWorld=Stored Integer
  Compare To Zero : simulink/Logic and Bit Operations/Compare To Zero  SystemSampleTime=-1  relop===  LogicOutDataTypeMode=uint8  ZeroCross=off
  Compare To Zero1 : simulink/Logic and Bit Operations/Compare To Zero  SystemSampleTime=-1  relop=~=  LogicOutDataTypeMode=boolean  ZeroCross=off
  Constant : Constant  Value=debouce  OutDataTypeStr=int32
  Constant1 : Constant  Value=mode  OutDataTypeStr=int32
  Data Type Conversion : DataTypeConversion  OutDataTypeStr=uint32
  Enabled Subsystem : Subsystem  TreatAsAtomicUnit=on
  Enabled Subsystem1 : Subsystem  TreatAsAtomicUnit=on
  Enabled Subsystem4 : Subsystem  TreatAsAtomicUnit=on
  Enabled Subsystem5 : Subsystem  TreatAsAtomicUnit=on
  Logical Operator : Logic  AllPortsSameDT=off  OutDataTypeStr=boolean
  Logical Operator1 : Logic  Inputs=3  AllPortsSameDT=off  OutDataTypeStr=boolean
  Logical Operator{2..3,5,7} (4 alike) : Logic  Operator=NOT  AllPortsSameDT=off  OutDataTypeStr=boolean
  Logical Operator4 : Logic  Operator=OR  AllPortsSameDT=off  OutDataTypeStr=boolean
  Logical Operator6 : Logic  AllPortsSameDT=off  OutDataTypeStr=boolean
  Memory{,1..3} (4 alike) : Memory  LinearizeMemory=on
  Multiport Switch : MultiPortSwitch
  Relational Operator : RelationalOperator  Operator=<  OutDataTypeStr=boolean
  Relational Operator1 : RelationalOperator  OutDataTypeStr=boolean  InputSameDT=on
  Out1 : Outport
  wires:
  Constant1/1 -> Multiport Switch/1
  Multiport Switch/1 -> Out1/1
  Data Type Conversion/1 -> Bitwise Operator/2
  Enabled Subsystem1/1(Out1) -> Multiport Switch/4
  Logical Operator6/1 -> Enabled Subsystem1/Enable, Multiport Switch/3
  In1/1 -> Compare To Zero/1
  Enabled Subsystem/1(Out1) -> Memory1/1
  Enabled Subsystem4/1(Out1) -> Memory/1
  Memory/1 -> Relational Operator/1, Add/1
  Memory1/1 -> Add/2, Relational Operator/2
  Compare To Zero/1 -> Logical Operator/2, Logical Operator3/1
  Logical Operator/1 -> Enabled Subsystem4/Enable
  Relational Operator/1 -> Logical Operator/1
  Add/1 -> Relational Operator1/1
  Constant/1 -> Data Type Conversion/1, Relational Operator1/2
  Logical Operator2/1 -> Logical Operator1/2
  Memory3/1 -> Logical Operator4/2, Logical Operator5/1
  Logical Operator5/1 -> Logical Operator1/3
  Logical Operator3/1 -> Logical Operator1/1
  Compare To Zero1/1 -> Memory3/1
  Bitwise Operator/1 -> Compare To Zero1/1
  Enabled Subsystem5/1(Out1) -> Bitwise Operator/1
  Logical Operator4/1 -> Enabled Subsystem5/Enable, Memory2/1, Logical Operator6/1
  Memory2/1 -> Logical Operator7/1
  Logical Operator7/1 -> Logical Operator6/2
  Relational Operator1/1 -> Multiport Switch/2, Logical Operator4/1, Logical Operator2/1
  Logical Operator1/1 -> Enabled Subsystem/Enable

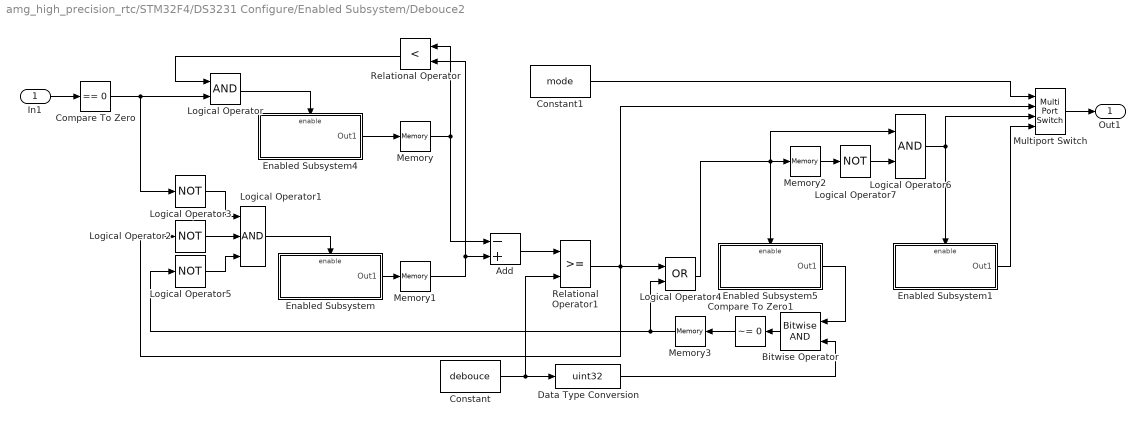
== system amg_high_precision_rtc/STM32F4/DS3231 Configure/Enabled Subsystem/Debouce2 ==
  In1 : Inport
  Add : Sum  Inputs=-+  OutDataTypeStr=int32
  Bitwise Operator : simulink/Logic and Bit Operations/Bitwise Operator  logicop=AND  UseBitMask=off  NumInputPorts=2  BitMask=debouce  BitMaskRealWorld=Stored Integer
  Compare To Zero : simulink/Logic and Bit Operations/Compare To Zero  SystemSampleTime=-1  relop===  LogicOutDataTypeMode=uint8  ZeroCross=off
  Compare To Zero1 : simulink/Logic and Bit Operations/Compare To Zero  SystemSampleTime=-1  relop=~=  LogicOutDataTypeMode=boolean  ZeroCross=off
  Constant : Constant  Value=debouce  OutDataTypeStr=int32
  Constant1 : Constant  Value=mode  OutDataTypeStr=int32
  Data Type Conversion : DataTypeConversion  OutDataTypeStr=uint32
  Enabled Subsystem : Subsystem  TreatAsAtomicUnit=on
  Enabled Subsystem1 : Subsystem  TreatAsAtomicUnit=on
  Enabled Subsystem4 : Subsystem  TreatAsAtomicUnit=on
  Enabled Subsystem5 : Subsystem  TreatAsAtomicUnit=on
  Logical Operator : Logic  AllPortsSameDT=off  OutDataTypeStr=boolean
  Logical Operator1 : Logic  Inputs=3  AllPortsSameDT=off  OutDataTypeStr=boolean
  Logical Operator{2..3,5,7} (4 alike) : Logic  Operator=NOT  AllPortsSameDT=off  OutDataTypeStr=boolean
  Logical Operator4 : Logic  Operator=OR  AllPortsSameDT=off  OutDataTypeStr=boolean
  Logical Operator6 : Logic  AllPortsSameDT=off  OutDataTypeStr=boolean
  Memory{,1..3} (4 alike) : Memory  LinearizeMemory=on
  Multiport Switch : MultiPortSwitch
  Relational Operator : RelationalOperator  Operator=<  OutDataTypeStr=boolean
  Relational Operator1 : RelationalOperator  OutDataTypeStr=boolean  InputSameDT=on
  Out1 : Outport
  wires:
  Constant1/1 -> Multiport Switch/1
  Multiport Switch/1 -> Out1/1
  Data Type Conversion/1 -> Bitwise Operator/2
  Enabled Subsystem1/1(Out1) -> Multiport Switch/4
  Logical Operator6/1 -> Enabled Subsystem1/Enable, Multiport Switch/3
  In1/1 -> Compare To Zero/1
  Enabled Subsystem/1(Out1) -> Memory1/1
  Enabled Subsystem4/1(Out1) -> Memory/1
  Memory/1 -> Relational Operator/1, Add/1
  Memory1/1 -> Add/2, Relational Operator/2
  Compare To Zero/1 -> Logical Operator/2, Logical Operator3/1
  Logical Operator/1 -> Enabled Subsystem4/Enable
  Relational Operator/1 -> Logical Operator/1
  Add/1 -> Relational Operator1/1
  Constant/1 -> Data Type Conversion/1, Relational Operator1/2
  Logical Operator2/1 -> Logical Operator1/2
  Memory3/1 -> Logical Operator4/2, Logical Operator5/1
  Logical Operator5/1 -> Logical Operator1/3
  Logical Operator3/1 -> Logical Operator1/1
  Compare To Zero1/1 -> Memory3/1
  Bitwise Operator/1 -> Compare To Zero1/1
  Enabled Subsystem5/1(Out1) -> Bitwise Operator/1
  Logical Operator4/1 -> Enabled Subsystem5/Enable, Memory2/1, Logical Operator6/1
  Memory2/1 -> Logical Operator7/1
  Logical Operator7/1 -> Logical Operator6/2
  Relational Operator1/1 -> Multiport Switch/2, Logical Operator4/1, Logical Operator2/1
  Logical Operator1/1 -> Enabled Subsystem/Enable

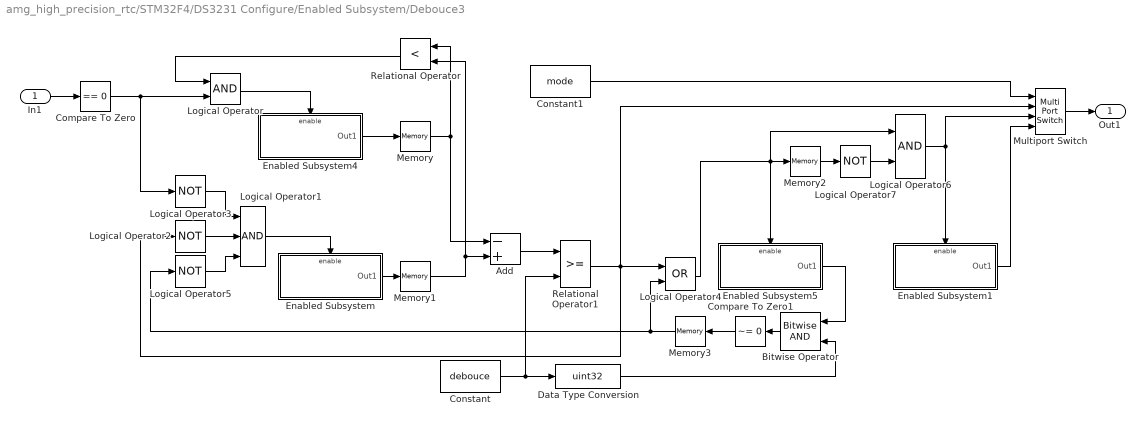
== system amg_high_precision_rtc/STM32F4/DS3231 Configure/Enabled Subsystem/Debouce3 ==
  In1 : Inport
  Add : Sum  Inputs=-+  OutDataTypeStr=int32
  Bitwise Operator : simulink/Logic and Bit Operations/Bitwise Operator  logicop=AND  UseBitMask=off  NumInputPorts=2  BitMask=debouce  BitMaskRealWorld=Stored Integer
  Compare To Zero : simulink/Logic and Bit Operations/Compare To Zero  SystemSampleTime=-1  relop===  LogicOutDataTypeMode=uint8  ZeroCross=off
  Compare To Zero1 : simulink/Logic and Bit Operations/Compare To Zero  SystemSampleTime=-1  relop=~=  LogicOutDataTypeMode=boolean  ZeroCross=off
  Constant : Constant  Value=debouce  OutDataTypeStr=int32
  Constant1 : Constant  Value=mode  OutDataTypeStr=int32
  Data Type Conversion : DataTypeConversion  OutDataTypeStr=uint32
  Enabled Subsystem : Subsystem  TreatAsAtomicUnit=on
  Enabled Subsystem1 : Subsystem  TreatAsAtomicUnit=on
  Enabled Subsystem4 : Subsystem  TreatAsAtomicUnit=on
  Enabled Subsystem5 : Subsystem  TreatAsAtomicUnit=on
  Logical Operator : Logic  AllPortsSameDT=off  OutDataTypeStr=boolean
  Logical Operator1 : Logic  Inputs=3  AllPortsSameDT=off  OutDataTypeStr=boolean
  Logical Operator{2..3,5,7} (4 alike) : Logic  Operator=NOT  AllPortsSameDT=off  OutDataTypeStr=boolean
  Logical Operator4 : Logic  Operator=OR  AllPortsSameDT=off  OutDataTypeStr=boolean
  Logical Operator6 : Logic  AllPortsSameDT=off  OutDataTypeStr=boolean
  Memory{,1..3} (4 alike) : Memory  LinearizeMemory=on
  Multiport Switch : MultiPortSwitch
  Relational Operator : RelationalOperator  Operator=<  OutDataTypeStr=boolean
  Relational Operator1 : RelationalOperator  OutDataTypeStr=boolean  InputSameDT=on
  Out1 : Outport
  wires:
  Constant1/1 -> Multiport Switch/1
  Multiport Switch/1 -> Out1/1
  Data Type Conversion/1 -> Bitwise Operator/2
  Enabled Subsystem1/1(Out1) -> Multiport Switch/4
  Logical Operator6/1 -> Enabled Subsystem1/Enable, Multiport Switch/3
  In1/1 -> Compare To Zero/1
  Enabled Subsystem/1(Out1) -> Memory1/1
  Enabled Subsystem4/1(Out1) -> Memory/1
  Memory/1 -> Relational Operator/1, Add/1
  Memory1/1 -> Add/2, Relational Operator/2
  Compare To Zero/1 -> Logical Operator/2, Logical Operator3/1
  Logical Operator/1 -> Enabled Subsystem4/Enable
  Relational Operator/1 -> Logical Operator/1
  Add/1 -> Relational Operator1/1
  Constant/1 -> Data Type Conversion/1, Relational Operator1/2
  Logical Operator2/1 -> Logical Operator1/2
  Memory3/1 -> Logical Operator4/2, Logical Operator5/1
  Logical Operator5/1 -> Logical Operator1/3
  Logical Operator3/1 -> Logical Operator1/1
  Compare To Zero1/1 -> Memory3/1
  Bitwise Operator/1 -> Compare To Zero1/1
  Enabled Subsystem5/1(Out1) -> Bitwise Operator/1
  Logical Operator4/1 -> Enabled Subsystem5/Enable, Memory2/1, Logical Operator6/1
  Memory2/1 -> Logical Operator7/1
  Logical Operator7/1 -> Logical Operator6/2
  Relational Operator1/1 -> Multiport Switch/2, Logical Operator4/1, Logical Operator2/1
  Logical Operator1/1 -> Enabled Subsystem/Enable

== system amg_high_precision_rtc/STM32F4/DS3231 Configure/Enabled Subsystem/Generate Mode ID ==
  note: # check unused state
  In1 : Inport
  Compare To Constant : simulink/Logic and Bit Operations/Compare To Constant  SystemSampleTime=-1  relop=>  const=5  LogicOutDataTypeMode=boolean  ZeroCross=off
  Enabled Subsystem2 : Subsystem  TreatAsAtomicUnit=on
  Logical Operator : Logic  Operator=OR  AllPortsSameDT=off  OutDataTypeStr=boolean
  Unit Delay : UnitDelay  SampleTime=-1
  Out1 : Outport
  wires:
  Enabled Subsystem2/1(Out1) -> Unit Delay/1, Out1/1
  Logical Operator/1 -> Enabled Subsystem2/Enable
  Compare To Constant/1 -> Logical Operator/1
  Unit Delay/1 -> Compare To Constant/1
  In1/1 -> Logical Operator/2

== system amg_high_precision_rtc/STM32F4/DS3231 Configure/Enabled Subsystem/Subsystem ==
  Up : Inport
  Down : Inport  Port=2
  SlvAddr : Inport  Port=3
  Adjust State : Inport  Port=4
  Enable : EnablePort  PropagateVarSize=During execution
  DS3231 Get Date : Subsystem  mask{blockfunction=date, module=1}
      mask prompts: blockfunction "Function"; module "I2C module"
      mask init:
      | amg_high_precision_rtc_callback('init');
      mask TypeOptions blockfunction: temp | time | date
      mask TypeOptions module: 1 | 2 | 3
      mask Callback module: amg_high_precision_rtc_callback('module');
      mask Display: text(0.5, 0.5, 'Port: I2C1','ver','middle','hor','center');port_label('input', 1,'SlvAddr');port_label('output', 1,'Status');port_label('output', 2,'Day(1-7)');port_label('output', 3,'Date(1-31)');port_label('output', 4,'Month(1-12)');port_label('output', 5,'Year(0-99)');
  DS3231 Get Time : Subsystem  mask{blockfunction=time, module=1}
      mask prompts: blockfunction "Function"; module "I2C module"
      mask init:
      | amg_high_precision_rtc_callback('init');
      mask TypeOptions blockfunction: temp | time | date
      mask TypeOptions module: 1 | 2 | 3
      mask Callback module: amg_high_precision_rtc_callback('module');
      mask Display: text(0.5, 0.5, 'Port: I2C1','ver','middle','hor','center');port_label('input', 1,'SlvAddr');port_label('output', 1,'Status');port_label('output', 2,'Hour(0-11/23)');port_label('output', 3,'Minute(0-59)');port_label('output', 4,'Second(0-59)');port_label('output', 5,'AM(0)/PM(1)');
  Enabled Subsystem : Subsystem  TreatAsAtomicUnit=on
  Logical Operator : Logic  AllPortsSameDT=off  OutDataTypeStr=boolean
  Terminator : Terminator
  Terminator1 : Terminator
  wires:
  DS3231 Get Date/4(Month) -> Enabled Subsystem/2(mm)
  DS3231 Get Date/5(Year) -> Enabled Subsystem/3(yy)
  SlvAddr/1 -> DS3231 Get Date/1(Slave Address), Enabled Subsystem/10(SlvAddr), DS3231 Get Time/1(Slave Address)
  DS3231 Get Date/2(Day) -> Terminator/1
  Adjust State/1 -> Enabled Subsystem/7(adjust state)
  Up/1 -> Enabled Subsystem/8(up)
  Down/1 -> Enabled Subsystem/9(down)
  DS3231 Get Time/2(Hour) -> Enabled Subsystem/4(hh)
  DS3231 Get Time/3(Minute) -> Enabled Subsystem/5(mi)
  DS3231 Get Time/4(Second) -> Enabled Subsystem/6(ss)
  DS3231 Get Date/3(Date) -> Enabled Subsystem/1(dd)
  DS3231 Get Time/5(AM/PM) -> Terminator1/1
  Logical Operator/1 -> Enabled Subsystem/Enable
  DS3231 Get Date/1(Status) -> Logical Operator/1
  DS3231 Get Time/1(Status) -> Logical Operator/2

== system amg_high_precision_rtc/STM32F4/DS3231 Get Date/Convert/Convert 1 ==
  In1 : Inport
  Add : Sum
  Constant : Constant  Value=10  OutDataTypeStr=uint8
  Extract Bits : simulink/Logic and Bit Operations/Extract Bits  SystemSampleTime=-1  bitsToExtract=Range of bits  numBits=8  bitIdxRange=[4 5]  outScalingMode=Treat bit field as an integer
  Extract Bits1 : simulink/Logic and Bit Operations/Extract Bits  SystemSampleTime=-1  bitsToExtract=Range of bits  numBits=8  bitIdxRange=[0 3]  outScalingMode=Treat bit field as an integer
  Product : Product  RndMeth=Zero
  Out1 : Outport
  wires:
  In1/1 -> Extract Bits/1, Extract Bits1/1
  Constant/1 -> Product/1
  Extract Bits/1 -> Product/2
  Product/1 -> Add/1
  Extract Bits1/1 -> Add/2
  Add/1 -> Out1/1

== system amg_high_precision_rtc/STM32F4/DS3231 Get Date/Convert/Convert 2 ==
  In1 : Inport
  Add : Sum
  Constant : Constant  Value=10  OutDataTypeStr=uint8
  Extract Bits : simulink/Logic and Bit Operations/Extract Bits  SystemSampleTime=-1  bitsToExtract=Range of bits  numBits=8  bitIdxRange=[4 4]  outScalingMode=Treat bit field as an integer
  Extract Bits1 : simulink/Logic and Bit Operations/Extract Bits  SystemSampleTime=-1  bitsToExtract=Range of bits  numBits=8  bitIdxRange=[0 3]  outScalingMode=Treat bit field as an integer
  Product : Product  RndMeth=Zero
  Out1 : Outport
  wires:
  Add/1 -> Out1/1
  Extract Bits1/1 -> Add/2
  Product/1 -> Add/1
  Extract Bits/1 -> Product/2
  Constant/1 -> Product/1
  In1/1 -> Extract Bits1/1, Extract Bits/1

== system amg_high_precision_rtc/STM32F4/DS3231 Get Date/Convert/Convert 3 ==
  In1 : Inport
  Add : Sum
  Constant : Constant  Value=10  OutDataTypeStr=uint8
  Extract Bits : simulink/Logic and Bit Operations/Extract Bits  SystemSampleTime=-1  bitsToExtract=Range of bits  numBits=8  bitIdxRange=[4 7]  outScalingMode=Treat bit field as an integer
  Extract Bits1 : simulink/Logic and Bit Operations/Extract Bits  SystemSampleTime=-1  bitsToExtract=Range of bits  numBits=8  bitIdxRange=[0 3]  outScalingMode=Treat bit field as an integer
  Product : Product  RndMeth=Zero
  Out1 : Outport
  wires:
  In1/1 -> Extract Bits/1, Extract Bits1/1
  Constant/1 -> Product/1
  Extract Bits/1 -> Product/2
  Product/1 -> Add/1
  Extract Bits1/1 -> Add/2
  Add/1 -> Out1/1
